simulink model "model_non_lineare2023b2"  (R2019b)
settings: Solver=VariableStepAuto  StartTime=0.0  StopTime=t_end  RelTol=1e-3
undefined symbols (not defined in the file or in its folder): Lc, Rtot
settings Model: Creator=Pronto all'uso  LastModifiedBy=Student
settings DebuggingCC: UnconnectedInputMsg=none  UnconnectedOutputMsg=none  UnconnectedLineMsg=none
settings ModelReferenceCC: EnableRefExpFcnMdlSchedulingChecks=off
settings RTWCC: Description=Generic Real-Time Target

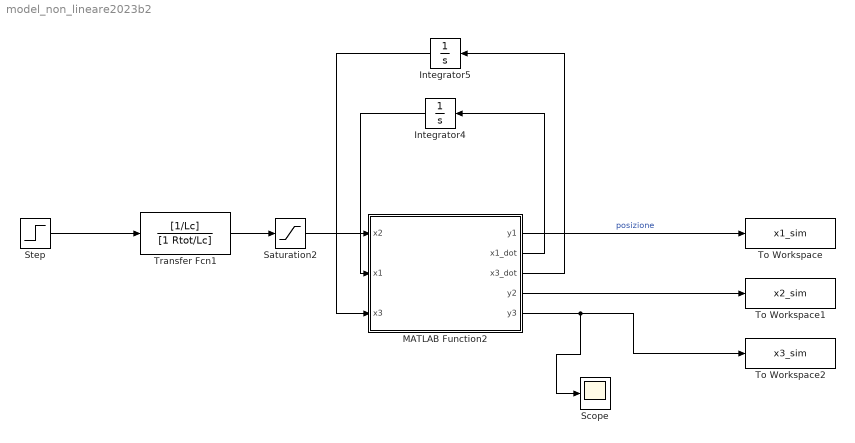
== system model_non_lineare2023b2 ==
  Integrator4 : Integrator
  Integrator5 : Integrator
  MATLAB Function2 : MATLAB Function  TreatAsAtomicUnit=on
  Saturation2 : Saturate  UpperLimit=3  LowerLimit=0
  Scope : Scope
  Step : Step  After=21  SampleTime=0.002
  To Workspace : ToWorkspace  VariableName=x1_sim  SampleTime=0.002
  To Workspace1 : ToWorkspace  VariableName=x2_sim  SampleTime=0.002
  To Workspace2 : ToWorkspace  VariableName=x3_sim  SampleTime=0.002
  Transfer Fcn1 : TransferFcn  Numerator=[1/Lc]  Denominator=[1 Rtot/Lc]
  wires:
  MATLAB Function2/2(x1_dot) -> Integrator4/1
  Integrator4/1 -> MATLAB Function2/2(x1)
  Saturation2/1 -> MATLAB Function2/1(x2)
  Integrator5/1 -> MATLAB Function2/3(x3)
  MATLAB Function2/3(x3_dot) -> Integrator5/1
  Transfer Fcn1/1 -> Saturation2/1
  Step/1 -> Transfer Fcn1/1
  MATLAB Function2/1(y1) -> To Workspace/1  "posizione"
  MATLAB Function2/4(y2) -> To Workspace1/1
  MATLAB Function2/5(y3) -> Scope/1, To Workspace2/1

== matlab function model_non_lineare2023b2/MATLAB Function2 ==
  data: y1 output; x2 input; x1_dot output; x1 input; x3 input; x3_dot output; y2 output; y3 output
function [y1,x1_dot, x3_dot, y2, y3] = fcn(x2, x1, x3)
    m = 0.0657;
    g = 9.81;
    k_mag = 2.4405e-05;
    Rtot = 9.7585;
    Lc = 0.3708;
    y0 = 0.012;
    
    x1_dot = x3;
    x3_dot = (k_mag/m)*(x2/(y0-x1))^2 - g;

    if x1 <= 0 && x3_dot < 0
        x1 = 0;
        x3 = 0;
        x3_dot = 0;
    end

    if x1 >= 0.012
        x1 = 0.012
        x3 = 0
    end
y1 = x1;
y2 = x2;
y3 = x3;
